simulink model "FADEC_Model1018"  (Simulink 8.3)
settings: Solver=ode3  StartTime=0.0  StopTime=100  FixedStep=0.02  RelTol=1e-3
undefined symbols (not defined in the file or in its folder): sigbuilder_block
settings Model: Creator=luzp  LastModifiedBy=luzp1
settings DataIOCC: SignalLoggingSaveFormat=Dataset
settings DebuggingCC: UnderspecifiedInitializationDetection=Simplified  StateNameClashWarn=none
settings GRTTargetCC: CombineOutputUpdateFcns=on  GRTInterface=off

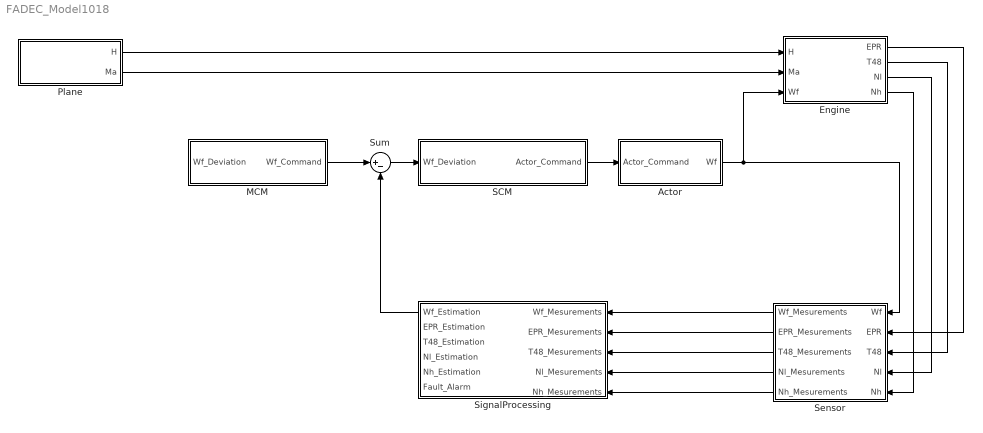
== system FADEC_Model1018 ==
  Actor : Subsystem  TreatAsAtomicUnit=on
  Engine : Subsystem  TreatAsAtomicUnit=on
  MCM : Subsystem  TreatAsAtomicUnit=on
  Plane : Subsystem  TreatAsAtomicUnit=on
  SCM : Subsystem  TreatAsAtomicUnit=on
  Sensor : Subsystem  TreatAsAtomicUnit=on
  SignalProcessing : Subsystem  TreatAsAtomicUnit=on
  Sum : Sum  Inputs=|+-
  wires:
  Plane/1(H) -> Engine/1(H)
  Plane/2(Ma) -> Engine/2(Ma)
  Actor/1(Wf) -> Engine/3(Wf), Sensor/1(Wf)
  Engine/1(EPR) -> Sensor/2(EPR)
  Engine/2(T48) -> Sensor/3(T48)
  Engine/3(Nl) -> Sensor/4(Nl)
  Engine/4(Nh) -> Sensor/5(Nh)
  Sensor/1(Wf_Mesurements) -> SignalProcessing/1(Wf_Mesurements)
  Sensor/2(EPR_Mesurements) -> SignalProcessing/2(EPR_Mesurements)
  Sensor/3(T48_Mesurements) -> SignalProcessing/3(T48_Mesurements)
  Sensor/4(Nl_Mesurements) -> SignalProcessing/4(Nl_Mesurements)
  Sensor/5(Nh_Mesurements) -> SignalProcessing/5(Nh_Mesurements)
  SignalProcessing/1(Wf_Estimation) -> Sum/2
  SCM/1(Actor_Command) -> Actor/1(Actor_Command)
  Sum/1 -> SCM/1(Wf_Deviation)
  MCM/1(Wf_Command) -> Sum/1

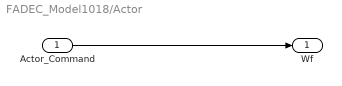
== system FADEC_Model1018/Actor ==
  Actor_Command : Inport
  Wf : Outport
  wires:
  Actor_Command/1 -> Wf/1

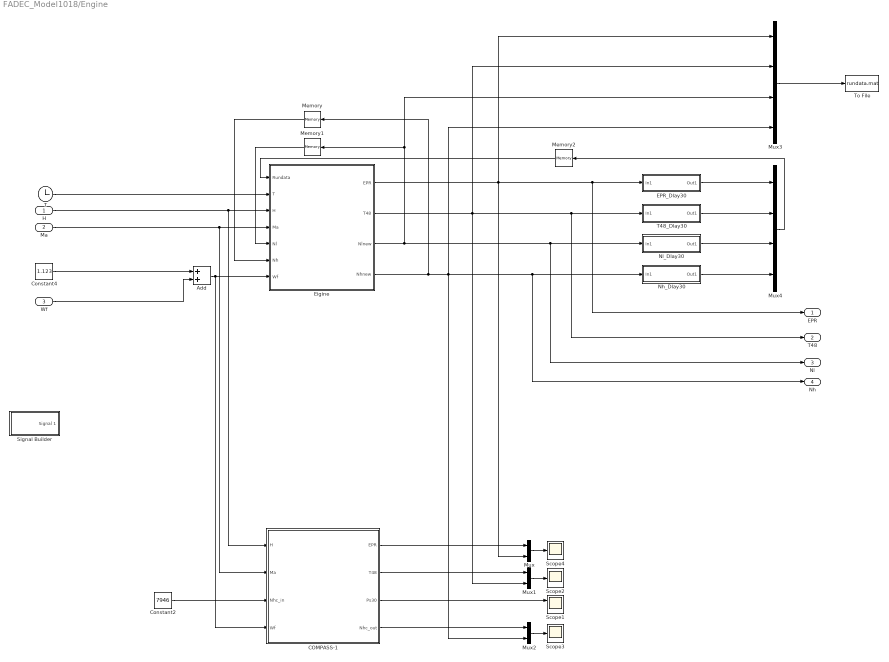
== system FADEC_Model1018/Engine ==
  H : Inport
  Ma : Inport  Port=2
  Wf : Inport  Port=3
  Add : Sum
  COMPASS-1 : Subsystem  TreatAsAtomicUnit=on
  Constant2 : Constant  Value=7946
  Constant4 : Constant  Value=1.123
  EPR_Dlay30 : Subsystem
  Eigine : MATLAB Function  TreatAsAtomicUnit=on
  Memory : Memory  X0=7503
  Memory1 : Memory  X0=1146
  Memory2 : Memory
  Mux : Mux  Inputs=2
  Mux1 : Mux  Inputs=2
  Mux2 : Mux  Inputs=2
  Mux3 : Mux
  Mux4 : Mux
  Nh_Dlay30 : Subsystem
  Nl_Dlay30 : Subsystem
  Scope1 : Scope  NumInputPorts=2
      settings: YMin=-5~-5  YMax=5~5
  Scope2 : Scope
      settings: SaveName=ScopeData2
  Scope3 : Scope
      settings: SaveName=ScopeData3
  Scope4 : Scope
  Signal Builder : Subsystem  Tag=STV Subsys  LoadFcn=sigbuilder_block('load');  StartFcn=sigbuilder_block('start');  StopFcn=sigbuilder_block('stop');  ClipboardFcn=sigbuilder_block('clipboard');  mask(Sigbuilder block){}
      mask help: Simulink:masks:SigbuilderBlock_MD
      mask init:
      | if ~strcmp(get_param(bdroot(gcbh),'SimulationStatus'),'stopped') tuvar = sigbuilder_block('maskInit'); end
      settings: CopyFcn=sigbuilder_block('copy');  DeleteFcn=sigbuilder_block('delete');  ModelCloseFcn=sigbuilder_block('modelClose');  PreSaveFcn=sigbuilder_block('preSave');  PauseFcn=sigbuilder_block('pause');  ContinueFcn=sigbuilder_block('continue');  NameChangeFcn=sigbuilder_block('namechange');  OpenFcn=sigbuilder_block('open',[40.5 6 1033.5 605.25 ]);  CloseFcn=sigbuilder_block('close');
      mask Display: plot(0, 0, 100, 100,[2, 2, 32, 32, 2], [68, 8, 8, 68, 68],[32, 2], [38, 38], [32, 19, 2],[53, 60, 44], [32, 17, 17, 2],[16, 16, 31, 31]);txt = getActiveGroup(gcbh);text(2, 100, txt,'verticalAlignment', 'top');
  T : Clock
  T48_Dlay30 : Subsystem
  To File : ToFile  Filename=rundata.mat  MatrixName=Sensor  SaveFormat=Timeseries
  EPR : Outport
  T48 : Outport  Port=2
  Nl : Outport  Port=3
  Nh : Outport  Port=4
  wires:
  H/1 -> COMPASS-1/1(H), Eigine/3(H)
  Ma/1 -> COMPASS-1/2(Ma), Eigine/4(Ma)
  Constant2/1 -> COMPASS-1/3(Nhc_in)
  Wf/1 -> Add/2
  COMPASS-1/2(T48) -> Mux1/1
  COMPASS-1/3(Ps30) -> Scope1/1
  COMPASS-1/4(Nhc_out) -> Mux2/1
  Eigine/3(Nlnew) -> Nl/1, Nl_Dlay30/1(In1), Mux3/3, Memory1/1
  Eigine/4(Nhnew) -> Nh/1, Nh_Dlay30/1(In1), Mux2/2, Mux3/4, Memory/1
  Eigine/2(T48) -> T48/1, T48_Dlay30/1(In1), Mux1/2, Mux3/2
  Memory1/1 -> Eigine/5(Nl)
  Memory/1 -> Eigine/6(Nh)
  Constant4/1 -> Add/1
  Add/1 -> Eigine/7(Wf), COMPASS-1/4(Wf)
  Mux1/1 -> Scope2/1
  Eigine/1(EPR) -> EPR/1, EPR_Dlay30/1(In1), Mux/2, Mux3/1
  Mux/1 -> Scope4/1
  COMPASS-1/1(EPR) -> Mux/1
  Mux2/1 -> Scope3/1
  Mux3/1 -> To File/1
  Nh_Dlay30/1(Out1) -> Mux4/4
  EPR_Dlay30/1(Out1) -> Mux4/1
  T48_Dlay30/1(Out1) -> Mux4/2
  Nl_Dlay30/1(Out1) -> Mux4/3
  Mux4/1 -> Memory2/1
  Memory2/1 -> Eigine/1(Rundata)
  T/1 -> Eigine/2(T)

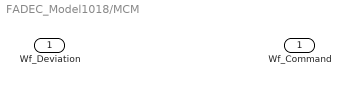
== system FADEC_Model1018/MCM ==
  Wf_Deviation : Inport
  Wf_Command : Outport

== system FADEC_Model1018/Plane ==
  H : Outport
  Ma : Outport  Port=2

== system FADEC_Model1018/SCM ==
  Wf_Deviation : Inport
  Actor_Command : Outport

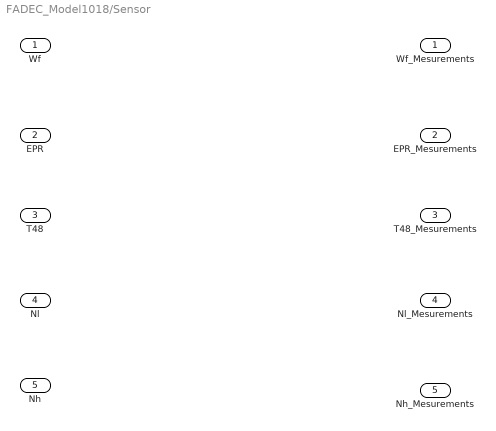
== system FADEC_Model1018/Sensor ==
  Wf : Inport
  EPR : Inport  Port=2
  T48 : Inport  Port=3
  Nl : Inport  Port=4
  Nh : Inport  Port=5
  Wf_Mesurements : Outport
  EPR_Mesurements : Outport  Port=2
  T48_Mesurements : Outport  Port=3
  Nl_Mesurements : Outport  Port=4
  Nh_Mesurements : Outport  Port=5

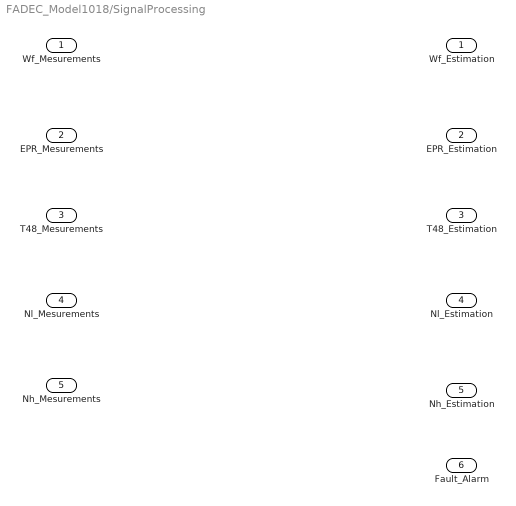
== system FADEC_Model1018/SignalProcessing ==
  Wf_Mesurements : Inport
  EPR_Mesurements : Inport  Port=2
  T48_Mesurements : Inport  Port=3
  Nl_Mesurements : Inport  Port=4
  Nh_Mesurements : Inport  Port=5
  Wf_Estimation : Outport
  EPR_Estimation : Outport  Port=2
  T48_Estimation : Outport  Port=3
  Nl_Estimation : Outport  Port=4
  Nh_Estimation : Outport  Port=5
  Fault_Alarm : Outport  Port=6

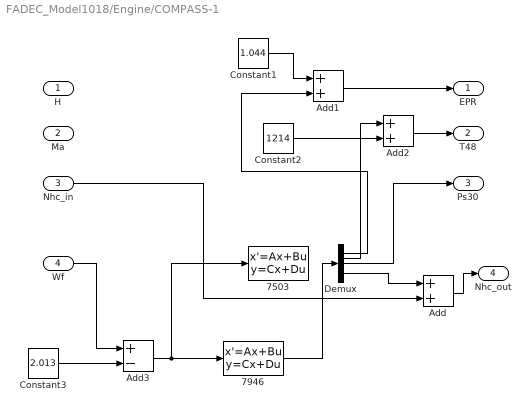
== system FADEC_Model1018/Engine/COMPASS-1 ==
  H : Inport
  Ma : Inport  Port=2
  Nhc_in : Inport  Port=3
  Wf : Inport  Port=4
  7503 : StateSpace  A=[-1.8470,0.7489;0.0996,-1.4302]  B=[305.0075;973.0158]  C=[0,0;0.0252,-0.1936;0.0054,0.0792;1,0;0,1]  D=[0.0093;423.5049;30.4577;0;0]  X0=0
  7946 : StateSpace  A=[-2.1668,1.2163;0.5305,-2.7527]  B=[293.1481;867.6547]  C=[0,0.0001;0.0561,-0.3109;-0.0079,0.1363;1,0;0,1]  D=[0.0118;307.2016;26.4699;0;0]  X0=0
  Add : Sum
  Add1 : Sum
  Add2 : Sum
  Add3 : Sum  Inputs=+-
  Constant1 : Constant  Value=1.044
  Constant2 : Constant  Value=1214
  Constant3 : Constant  Value=2.013
  Demux : Demux  Outputs=5
  EPR : Outport
  T48 : Outport  Port=2
  Ps30 : Outport  Port=3
  Nhc_out : Outport  Port=4
  wires:
  Demux/3 -> Ps30/1
  Nhc_in/1 -> Add/2
  Demux/5 -> Add/1
  Add/1 -> Nhc_out/1
  Constant1/1 -> Add1/1
  Add1/1 -> EPR/1
  Demux/1 -> Add1/2
  Add2/1 -> T48/1
  Demux/2 -> Add2/1
  Constant2/1 -> Add2/2
  Add3/1 -> 7503/1, 7946/1
  Wf/1 -> Add3/1
  Constant3/1 -> Add3/2
  7946/1 -> Demux/1

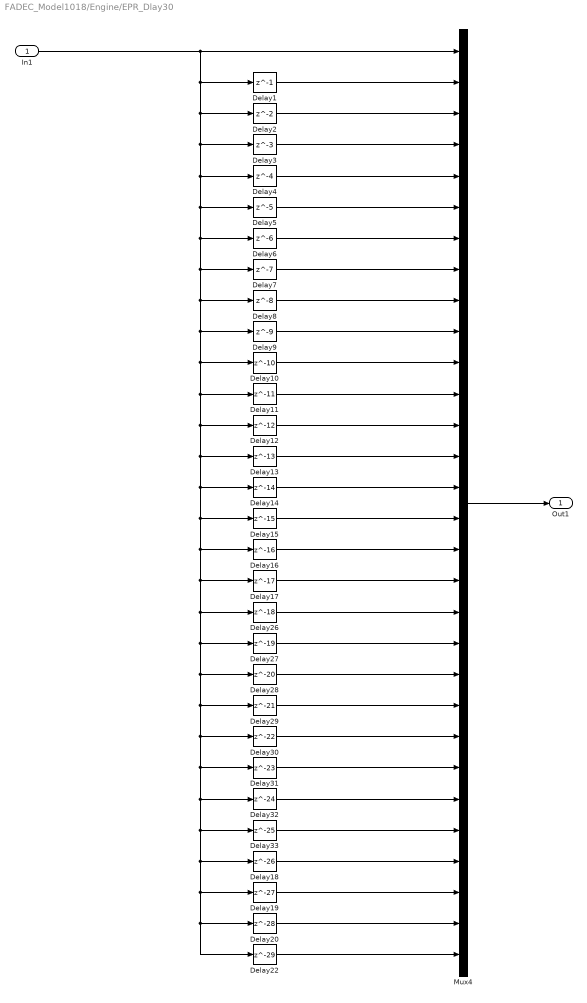
== system FADEC_Model1018/Engine/EPR_Dlay30 ==
  In1 : Inport
  Delay1 : Delay  DelayLength=1  InitialCondition=0
  Delay10 : Delay  DelayLength=10  InitialCondition=0
  Delay11 : Delay  DelayLength=11  InitialCondition=0
  Delay12 : Delay  DelayLength=12  InitialCondition=0
  Delay13 : Delay  DelayLength=13  InitialCondition=0
  Delay14 : Delay  DelayLength=14  InitialCondition=0
  Delay15 : Delay  DelayLength=15  InitialCondition=0
  Delay16 : Delay  DelayLength=16  InitialCondition=0
  Delay17 : Delay  DelayLength=17  InitialCondition=0
  Delay18 : Delay  DelayLength=26  InitialCondition=0
  Delay19 : Delay  DelayLength=27  InitialCondition=0
  Delay2 : Delay  InitialCondition=0
  Delay20 : Delay  DelayLength=28  InitialCondition=0
  Delay22 : Delay  DelayLength=29  InitialCondition=0
  Delay26 : Delay  DelayLength=18  InitialCondition=0
  Delay27 : Delay  DelayLength=19  InitialCondition=0
  Delay28 : Delay  DelayLength=20  InitialCondition=0
  Delay29 : Delay  DelayLength=21  InitialCondition=0
  Delay3 : Delay  DelayLength=3  InitialCondition=0
  Delay30 : Delay  DelayLength=22  InitialCondition=0
  Delay31 : Delay  DelayLength=23  InitialCondition=0
  Delay32 : Delay  DelayLength=24  InitialCondition=0
  Delay33 : Delay  DelayLength=25  InitialCondition=0
  Delay4 : Delay  DelayLength=4  InitialCondition=0
  Delay5 : Delay  DelayLength=5  InitialCondition=0
  Delay6 : Delay  DelayLength=6  InitialCondition=0
  Delay7 : Delay  DelayLength=7  InitialCondition=0
  Delay8 : Delay  DelayLength=8  InitialCondition=0
  Delay9 : Delay  DelayLength=9  InitialCondition=0
  Mux4 : Mux  Inputs=30
  Out1 : Outport
  wires:
  Delay1/1 -> Mux4/2
  Delay2/1 -> Mux4/3
  Delay3/1 -> Mux4/4
  Delay4/1 -> Mux4/5
  Delay5/1 -> Mux4/6
  Delay6/1 -> Mux4/7
  Delay7/1 -> Mux4/8
  Delay8/1 -> Mux4/9
  Delay9/1 -> Mux4/10
  Delay10/1 -> Mux4/11
  Delay11/1 -> Mux4/12
  Delay12/1 -> Mux4/13
  Delay13/1 -> Mux4/14
  Delay14/1 -> Mux4/15
  Delay15/1 -> Mux4/16
  Delay16/1 -> Mux4/17
  Delay17/1 -> Mux4/18
  Delay26/1 -> Mux4/19
  Delay27/1 -> Mux4/20
  Delay28/1 -> Mux4/21
  Delay29/1 -> Mux4/22
  Delay30/1 -> Mux4/23
  Delay31/1 -> Mux4/24
  Delay32/1 -> Mux4/25
  Delay33/1 -> Mux4/26
  Delay18/1 -> Mux4/27
  Delay19/1 -> Mux4/28
  Delay20/1 -> Mux4/29
  Delay22/1 -> Mux4/30
  In1/1 -> Mux4/1, Delay2/1, Delay14/1, Delay15/1, Delay16/1, Delay26/1, Delay27/1, Delay28/1, Delay29/1, Delay30/1, Delay31/1, Delay32/1, Delay33/1, Delay18/1, Delay19/1, Delay20/1, Delay22/1, Delay17/1, Delay13/1, Delay12/1, Delay11/1, Delay10/1, Delay9/1, Delay8/1, Delay7/1, Delay6/1, Delay5/1, Delay4/1, Delay3/1, Delay1/1
  Mux4/1 -> Out1/1

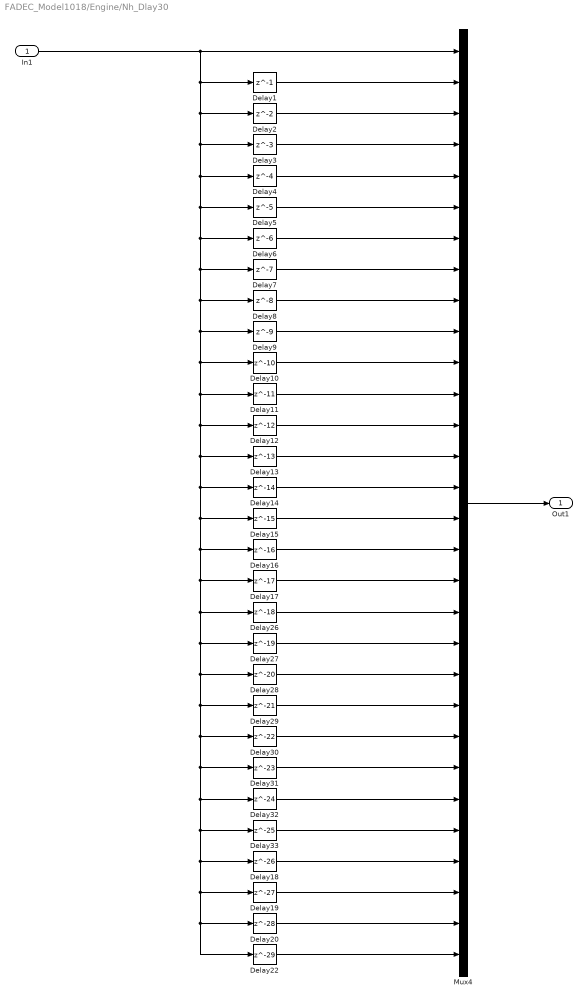
== system FADEC_Model1018/Engine/Nh_Dlay30 ==
  In1 : Inport
  Delay1 : Delay  DelayLength=1  InitialCondition=0
  Delay10 : Delay  DelayLength=10  InitialCondition=0
  Delay11 : Delay  DelayLength=11  InitialCondition=0
  Delay12 : Delay  DelayLength=12  InitialCondition=0
  Delay13 : Delay  DelayLength=13  InitialCondition=0
  Delay14 : Delay  DelayLength=14  InitialCondition=0
  Delay15 : Delay  DelayLength=15  InitialCondition=0
  Delay16 : Delay  DelayLength=16  InitialCondition=0
  Delay17 : Delay  DelayLength=17  InitialCondition=0
  Delay18 : Delay  DelayLength=26  InitialCondition=0
  Delay19 : Delay  DelayLength=27  InitialCondition=0
  Delay2 : Delay  InitialCondition=0
  Delay20 : Delay  DelayLength=28  InitialCondition=0
  Delay22 : Delay  DelayLength=29  InitialCondition=0
  Delay26 : Delay  DelayLength=18  InitialCondition=0
  Delay27 : Delay  DelayLength=19  InitialCondition=0
  Delay28 : Delay  DelayLength=20  InitialCondition=0
  Delay29 : Delay  DelayLength=21  InitialCondition=0
  Delay3 : Delay  DelayLength=3  InitialCondition=0
  Delay30 : Delay  DelayLength=22  InitialCondition=0
  Delay31 : Delay  DelayLength=23  InitialCondition=0
  Delay32 : Delay  DelayLength=24  InitialCondition=0
  Delay33 : Delay  DelayLength=25  InitialCondition=0
  Delay4 : Delay  DelayLength=4  InitialCondition=0
  Delay5 : Delay  DelayLength=5  InitialCondition=0
  Delay6 : Delay  DelayLength=6  InitialCondition=0
  Delay7 : Delay  DelayLength=7  InitialCondition=0
  Delay8 : Delay  DelayLength=8  InitialCondition=0
  Delay9 : Delay  DelayLength=9  InitialCondition=0
  Mux4 : Mux  Inputs=30
  Out1 : Outport
  wires:
  Delay1/1 -> Mux4/2
  Delay2/1 -> Mux4/3
  Delay3/1 -> Mux4/4
  Delay4/1 -> Mux4/5
  Delay5/1 -> Mux4/6
  Delay6/1 -> Mux4/7
  Delay7/1 -> Mux4/8
  Delay8/1 -> Mux4/9
  Delay9/1 -> Mux4/10
  Delay10/1 -> Mux4/11
  Delay11/1 -> Mux4/12
  Delay12/1 -> Mux4/13
  Delay13/1 -> Mux4/14
  Delay14/1 -> Mux4/15
  Delay15/1 -> Mux4/16
  Delay16/1 -> Mux4/17
  Delay17/1 -> Mux4/18
  Delay26/1 -> Mux4/19
  Delay27/1 -> Mux4/20
  Delay28/1 -> Mux4/21
  Delay29/1 -> Mux4/22
  Delay30/1 -> Mux4/23
  Delay31/1 -> Mux4/24
  Delay32/1 -> Mux4/25
  Delay33/1 -> Mux4/26
  Delay18/1 -> Mux4/27
  Delay19/1 -> Mux4/28
  Delay20/1 -> Mux4/29
  Delay22/1 -> Mux4/30
  In1/1 -> Mux4/1, Delay2/1, Delay14/1, Delay15/1, Delay16/1, Delay26/1, Delay27/1, Delay28/1, Delay29/1, Delay30/1, Delay31/1, Delay32/1, Delay33/1, Delay18/1, Delay19/1, Delay20/1, Delay22/1, Delay17/1, Delay13/1, Delay12/1, Delay11/1, Delay10/1, Delay9/1, Delay8/1, Delay7/1, Delay6/1, Delay5/1, Delay4/1, Delay3/1, Delay1/1
  Mux4/1 -> Out1/1

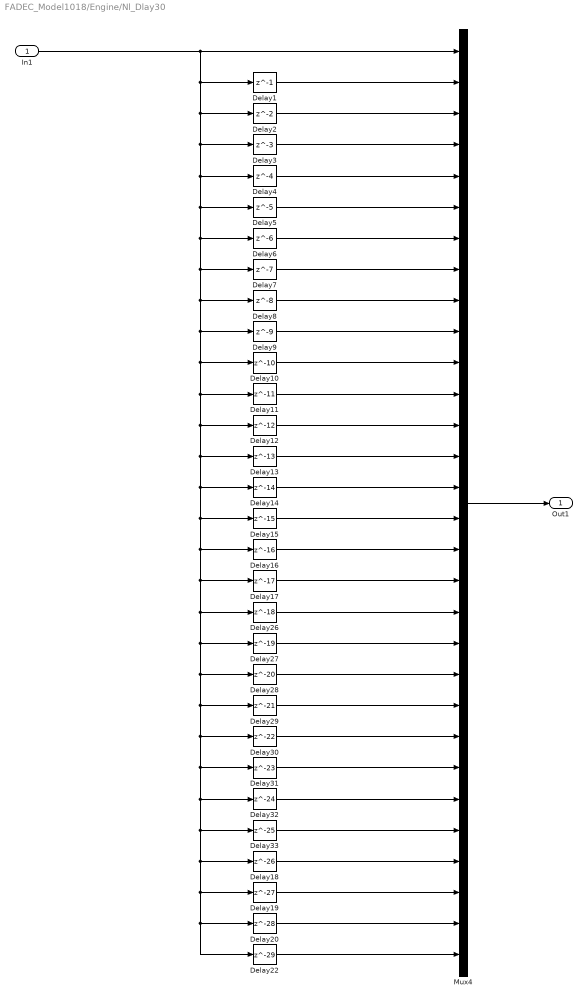
== system FADEC_Model1018/Engine/Nl_Dlay30 ==
  In1 : Inport
  Delay1 : Delay  DelayLength=1  InitialCondition=0
  Delay10 : Delay  DelayLength=10  InitialCondition=0
  Delay11 : Delay  DelayLength=11  InitialCondition=0
  Delay12 : Delay  DelayLength=12  InitialCondition=0
  Delay13 : Delay  DelayLength=13  InitialCondition=0
  Delay14 : Delay  DelayLength=14  InitialCondition=0
  Delay15 : Delay  DelayLength=15  InitialCondition=0
  Delay16 : Delay  DelayLength=16  InitialCondition=0
  Delay17 : Delay  DelayLength=17  InitialCondition=0
  Delay18 : Delay  DelayLength=26  InitialCondition=0
  Delay19 : Delay  DelayLength=27  InitialCondition=0
  Delay2 : Delay  InitialCondition=0
  Delay20 : Delay  DelayLength=28  InitialCondition=0
  Delay22 : Delay  DelayLength=29  InitialCondition=0
  Delay26 : Delay  DelayLength=18  InitialCondition=0
  Delay27 : Delay  DelayLength=19  InitialCondition=0
  Delay28 : Delay  DelayLength=20  InitialCondition=0
  Delay29 : Delay  DelayLength=21  InitialCondition=0
  Delay3 : Delay  DelayLength=3  InitialCondition=0
  Delay30 : Delay  DelayLength=22  InitialCondition=0
  Delay31 : Delay  DelayLength=23  InitialCondition=0
  Delay32 : Delay  DelayLength=24  InitialCondition=0
  Delay33 : Delay  DelayLength=25  InitialCondition=0
  Delay4 : Delay  DelayLength=4  InitialCondition=0
  Delay5 : Delay  DelayLength=5  InitialCondition=0
  Delay6 : Delay  DelayLength=6  InitialCondition=0
  Delay7 : Delay  DelayLength=7  InitialCondition=0
  Delay8 : Delay  DelayLength=8  InitialCondition=0
  Delay9 : Delay  DelayLength=9  InitialCondition=0
  Mux4 : Mux  Inputs=30
  Out1 : Outport
  wires:
  Delay1/1 -> Mux4/2
  Delay2/1 -> Mux4/3
  Delay3/1 -> Mux4/4
  Delay4/1 -> Mux4/5
  Delay5/1 -> Mux4/6
  Delay6/1 -> Mux4/7
  Delay7/1 -> Mux4/8
  Delay8/1 -> Mux4/9
  Delay9/1 -> Mux4/10
  Delay10/1 -> Mux4/11
  Delay11/1 -> Mux4/12
  Delay12/1 -> Mux4/13
  Delay13/1 -> Mux4/14
  Delay14/1 -> Mux4/15
  Delay15/1 -> Mux4/16
  Delay16/1 -> Mux4/17
  Delay17/1 -> Mux4/18
  Delay26/1 -> Mux4/19
  Delay27/1 -> Mux4/20
  Delay28/1 -> Mux4/21
  Delay29/1 -> Mux4/22
  Delay30/1 -> Mux4/23
  Delay31/1 -> Mux4/24
  Delay32/1 -> Mux4/25
  Delay33/1 -> Mux4/26
  Delay18/1 -> Mux4/27
  Delay19/1 -> Mux4/28
  Delay20/1 -> Mux4/29
  Delay22/1 -> Mux4/30
  In1/1 -> Mux4/1, Delay2/1, Delay14/1, Delay15/1, Delay16/1, Delay26/1, Delay27/1, Delay28/1, Delay29/1, Delay30/1, Delay31/1, Delay32/1, Delay33/1, Delay18/1, Delay19/1, Delay20/1, Delay22/1, Delay17/1, Delay13/1, Delay12/1, Delay11/1, Delay10/1, Delay9/1, Delay8/1, Delay7/1, Delay6/1, Delay5/1, Delay4/1, Delay3/1, Delay1/1
  Mux4/1 -> Out1/1

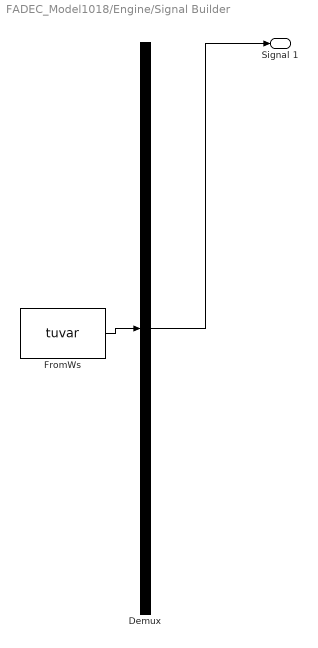
== system FADEC_Model1018/Engine/Signal Builder ==
  Demux : Demux  Tag=STV Demux  Outputs=1
  FromWs : FromWorkspace  Tag=STV FromWs  VariableName=tuvar  SampleTime=0  SigBuilderData=DataTag0  VnvData=DataTag1
      SigBuilderData=|
      | common.afterFinalStr = 'Extrapolate'
      | common.sampleTime = 0
      | dataSet.timeRange = [0 100]
      | dataSet.name = 'Group 1'
      | sbobj.Groups.Name = 'Group 1'
      | sbobj.Groups.Signals.Name = 'Signal 1'
      | sbobj.Groups.Signals.XData = [0 40 40 50 50 60 60 70 70 80 80 90 90 100]
      | sbobj.Groups.Signals.YData = [0 0 0.1 0.1 0.2 0.1998925 1 1 0.2 0.2 0.1 0.1 0 0]
      | sbobj.Groups.TimeRange = [0 100]
  Signal 1 : Outport  Tag=STV Outport
  wires:
  Demux/1 -> Signal 1/1
  FromWs/1 -> Demux/1

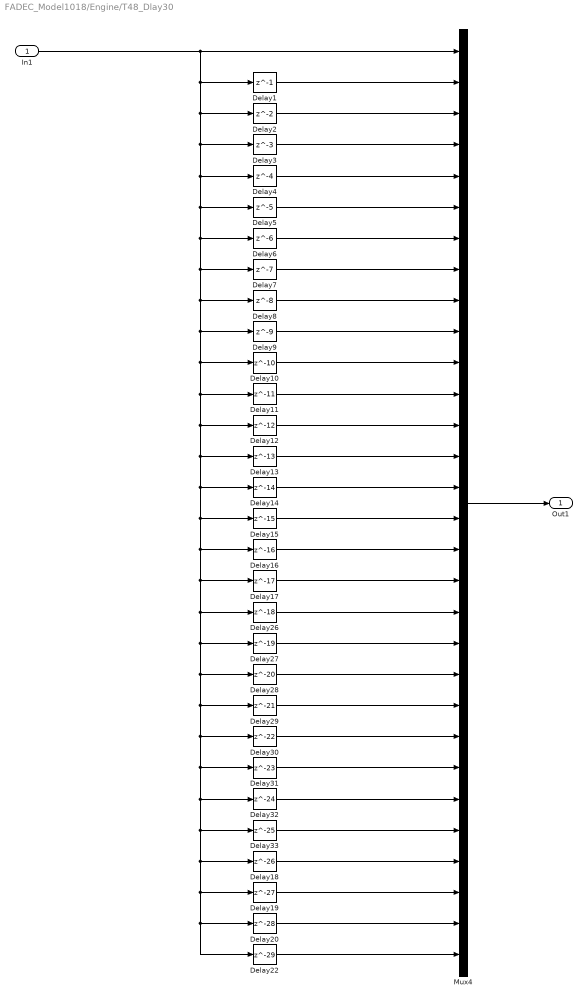
== system FADEC_Model1018/Engine/T48_Dlay30 ==
  In1 : Inport
  Delay1 : Delay  DelayLength=1  InitialCondition=0
  Delay10 : Delay  DelayLength=10  InitialCondition=0
  Delay11 : Delay  DelayLength=11  InitialCondition=0
  Delay12 : Delay  DelayLength=12  InitialCondition=0
  Delay13 : Delay  DelayLength=13  InitialCondition=0
  Delay14 : Delay  DelayLength=14  InitialCondition=0
  Delay15 : Delay  DelayLength=15  InitialCondition=0
  Delay16 : Delay  DelayLength=16  InitialCondition=0
  Delay17 : Delay  DelayLength=17  InitialCondition=0
  Delay18 : Delay  DelayLength=26  InitialCondition=0
  Delay19 : Delay  DelayLength=27  InitialCondition=0
  Delay2 : Delay  InitialCondition=0
  Delay20 : Delay  DelayLength=28  InitialCondition=0
  Delay22 : Delay  DelayLength=29  InitialCondition=0
  Delay26 : Delay  DelayLength=18  InitialCondition=0
  Delay27 : Delay  DelayLength=19  InitialCondition=0
  Delay28 : Delay  DelayLength=20  InitialCondition=0
  Delay29 : Delay  DelayLength=21  InitialCondition=0
  Delay3 : Delay  DelayLength=3  InitialCondition=0
  Delay30 : Delay  DelayLength=22  InitialCondition=0
  Delay31 : Delay  DelayLength=23  InitialCondition=0
  Delay32 : Delay  DelayLength=24  InitialCondition=0
  Delay33 : Delay  DelayLength=25  InitialCondition=0
  Delay4 : Delay  DelayLength=4  InitialCondition=0
  Delay5 : Delay  DelayLength=5  InitialCondition=0
  Delay6 : Delay  DelayLength=6  InitialCondition=0
  Delay7 : Delay  DelayLength=7  InitialCondition=0
  Delay8 : Delay  DelayLength=8  InitialCondition=0
  Delay9 : Delay  DelayLength=9  InitialCondition=0
  Mux4 : Mux  Inputs=30
  Out1 : Outport
  wires:
  Delay1/1 -> Mux4/2
  Delay2/1 -> Mux4/3
  Delay3/1 -> Mux4/4
  Delay4/1 -> Mux4/5
  Delay5/1 -> Mux4/6
  Delay6/1 -> Mux4/7
  Delay7/1 -> Mux4/8
  Delay8/1 -> Mux4/9
  Delay9/1 -> Mux4/10
  Delay10/1 -> Mux4/11
  Delay11/1 -> Mux4/12
  Delay12/1 -> Mux4/13
  Delay13/1 -> Mux4/14
  Delay14/1 -> Mux4/15
  Delay15/1 -> Mux4/16
  Delay16/1 -> Mux4/17
  Delay17/1 -> Mux4/18
  Delay26/1 -> Mux4/19
  Delay27/1 -> Mux4/20
  Delay28/1 -> Mux4/21
  Delay29/1 -> Mux4/22
  Delay30/1 -> Mux4/23
  Delay31/1 -> Mux4/24
  Delay32/1 -> Mux4/25
  Delay33/1 -> Mux4/26
  Delay18/1 -> Mux4/27
  Delay19/1 -> Mux4/28
  Delay20/1 -> Mux4/29
  Delay22/1 -> Mux4/30
  In1/1 -> Mux4/1, Delay2/1, Delay14/1, Delay15/1, Delay16/1, Delay26/1, Delay27/1, Delay28/1, Delay29/1, Delay30/1, Delay31/1, Delay32/1, Delay33/1, Delay18/1, Delay19/1, Delay20/1, Delay22/1, Delay17/1, Delay13/1, Delay12/1, Delay11/1, Delay10/1, Delay9/1, Delay8/1, Delay7/1, Delay6/1, Delay5/1, Delay4/1, Delay3/1, Delay1/1
  Mux4/1 -> Out1/1

== matlab function Engine/Eigine ==
  settings: updateMethod=DISCRETE  sampleTime=0.02
  data: Rundata input double; T input double; H input double; Ma input double; EPR output double; Nl input double; Nh input double; T48 output double; Wf input double; Nlnew output double; Nhnew output double
function [EPR,T48,Nlnew,Nhnew]   = CompassModel(Rundata,T,H,Ma,Nl,Nh,Wf)
%#codegen
% coder.extrinsic('load');
% coder.extrinsic('evalin');
% evalin('Model','load（''matlab.mat''）');

%参数设置
Simulationstep=0.02;%仿真间隔，s
P_steptime=0.1;%参数更新频率,s


FC=[
-3.8557	1.4467	0.469	-4.7081	230.6739	653.5547	0.0000	0.0002	-0.0573	-0.3224	0.0514	0.1912	0.0236	146.37	20.1147;
-3.6284	1.5373	0.9017	-4.6475	247.3701	685.2015	0.0000	0.0002	0.0058	-0.348	0.0178	0.1947	0.0204	167.9945	20.9823;
-3.3384	1.4517	0.8547	-4.2881	262.2267	773.8465	0.0000	0.0001	0.0807	-0.3435	0.0036	0.1557	0.0145	236.438	22.7029;
-2.6591	1.3162	0.5251	-3.2409	274.6438	814.375	0	0.0001	0.0807	-0.3435	-0.0067	0.1558	0.0145	236.438	24.2831;
-2.1668	1.2163	0.5305	-2.7527	293.1481	867.6547	0.0000	0.0001	0.0561	-0.3109	-0.0079	0.1363	0.0118	307.2016	26.4699;
-1.847	0.7489	0.0996	-1.4302	305.0075	973.0158	0.0000	0.0000	0.0252	-0.1936	0.0054	0.0792	0.0093	423.5049	30.4577
];
%FC_IN:14个状态，8个参数：高度、马赫数、燃油流量、风扇转速、高压转速、增压比、排气温度、净推力
FC_IN=[
0	0	6.835	2388	9051	1.3	2072	86336
0	0	5.511	2224	8837	1.227	1941	71652
0	0	4.254	2028	8592	1.165	1792	57181
0	0	3.075	1797	8299	1.114	1623	42562
0	0	2.013	1497	7946	1.073	1433	28016
0	0	1.123	1146	7503	1.044	1214	13448
];
P_ABCD=zeros(1,15);
Nhc=7503/sqrt(calTtotal(H,Ma)/288.15);


NumNh=round(rem(T/Simulationstep,P_steptime/Simulationstep));
if T>P_steptime
Nhc=Rundata(91+NumNh)/sqrt(calTtotal(H,Ma)/288.15);
end
% Nhc=Sensor.data(t/0.02+1,4)/sqrt(calTtotal(H,Ma)/288.15);
%依次插值得到矩阵方程系数
for i=1:15
    P_ABCD(i)=interp1(FC_IN(:,5),FC(:,i),Nhc,'spline');
end

%确定当前矩阵方程对应的发动机状态基准点
Steady_Condition=zeros(1,5);
for i=1:5
    Steady_Condition(i)=interp1(FC_IN(:,5),FC_IN(:,2+i),Nhc,'spline');
end
Ac=[P_ABCD(1),P_ABCD(2);P_ABCD(3),P_ABCD(4)];
Bc=[P_ABCD(5);P_ABCD(6)];
C=[P_ABCD(7),P_ABCD(8);P_ABCD(9),P_ABCD(10);P_ABCD(11),P_ABCD(12)];
D=[P_ABCD(13);P_ABCD(14);P_ABCD(15)];
% 状态方程离散化
[m,n] = size(Ac); %#ok<ASGLU>
[m,nb] = size(Bc); %#ok<ASGLU>
timestep=Simulationstep;
s = expm([[Ac Bc]*timestep; zeros(nb,n+nb)]);
A = s(1:n,1:n);
B = s(1:n,n+1:n+nb);


%计算delta
dx0=[Nl-Steady_Condition(2);Nh-Steady_Condition(3)];
du=Wf-Steady_Condition(1);
dxnew=zeros(2,1);
dxnew=A*dx0+B*du;
dy=zeros(3,1);
dy=C*dx0+D*du;
Nlnew=dxnew(1,1)+Steady_Condition(2);Nhnew=dxnew(2,1)+Steady_Condition(3);
EPR=dy(1,1)+Steady_Condition(4);T48=dy(2,1)+Steady_Condition(5);%Ps30=dy(3,1);
% Steady_Condition
